simulink model "example19teen"  (R2023b)
settings: Solver=VariableStepAuto  StartTime=0.0  StopTime=10.0  RelTol=1e-3
settings Model: Creator=ray  LastModifiedBy=ray

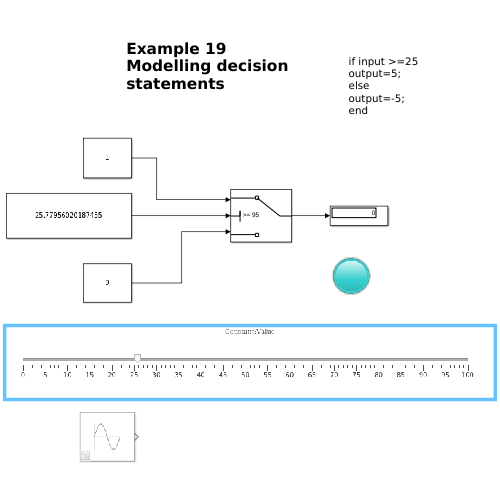
[thumbnail: Simulink's stored preview of the top-level diagram]
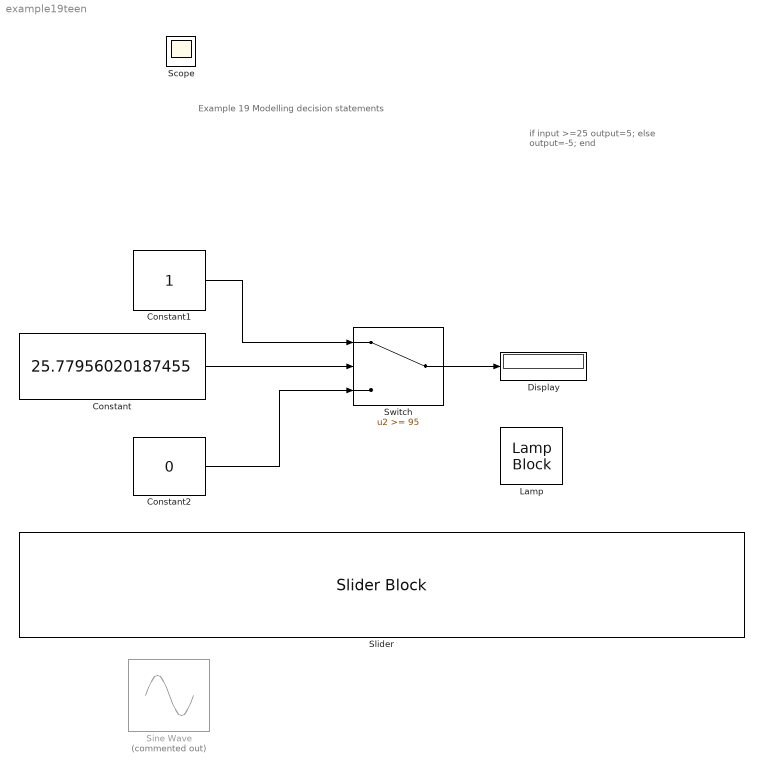
== system example19teen ==
  note: if input >=25
      | output=5;
      | else
      | output=-5;
      | end
  note: Example 19
      | Modelling decision
      | statements
  Constant : Constant  Value=25.77956020187455
  Constant1 : Constant
  Constant2 : Constant  Value=0
  Display : Display
  Lamp : LampBlock  LabelPosition=Hide
  Sine Wave : Sin  Commented=on  SampleTime=0
  Slider : SliderBlock  TickInterval=5
  Switch : Switch  Threshold=95  SaturateOnIntegerOverflow=off  InputSameDT=off
  Scope : Scope
  wires:
  Constant/1 -> Switch/2
  Constant1/1 -> Switch/1
  Constant2/1 -> Switch/3
  Switch/1 -> Display/1
